simulink model "AprilTagPlant"  (R2024b)
settings: Solver=ode4  StartTime=0.0  StopTime=Tsim  FixedStep=0.005  RelTol=1e-3
values from neighbouring files (symbols this model uses):
  Caf = 20    [AprilTagVehicleSetup.m]
  Car = 20    [AprilTagVehicleSetup.m]
  circle_dir = 1    [AprilTagVehicleSetup.m]
  delta_corr_max_rad = deg2rad(20)    [AprilTagVehicleSetup.m]
  delta_max_rad = deg2rad(25)    [AprilTagVehicleSetup.m]
  delta_test_rad = deg2rad(8)    [AprilTagVehicleSetup.m]
  dist_psi_step_amp_rad = deg2rad(10)    [AprilTagVehicleSetup.m]
  dist_psi_step_time_s = 9.0    (= 9)    [AprilTagVehicleSetup.m]
  dist_x_step_amp_m = 0.10    (= 0.1)    [AprilTagVehicleSetup.m]
  dist_x_step_time_s = 5.0    (= 5)    [AprilTagVehicleSetup.m]
  dist_y_step_time_s = 7.0    (= 7)    [AprilTagVehicleSetup.m]
  Jz = 0.015    [AprilTagVehicleSetup.m]
  Kd_radius_pid = 0.0    (= 0)    [AprilTagVehicleSetup.m]
  Ki_radius_pid = 0.0    (= 0)    [AprilTagVehicleSetup.m]
  Kp_radius_pid = 0.6    [AprilTagVehicleSetup.m]
  L = 0.26    [AprilTagVehicleSetup.m]
  lf = 0.13    [AprilTagVehicleSetup.m]
  lr = 0.13    [AprilTagVehicleSetup.m]
  m = 1.5    [AprilTagVehicleSetup.m]
  noise_psi_std_rad = deg2rad(0.5)    [AprilTagVehicleSetup.m]
  noise_x_std_m = 0.005    [AprilTagVehicleSetup.m]
  noise_y_std_m = 0.005    [AprilTagVehicleSetup.m]
  psi0_rad = pi/2 - deg2rad(45)    [AprilTagVehicleSetup.m]
  psi_offset_max_rad = deg2rad(30)    [AprilTagVehicleSetup.m]
  r0_radps = 0.0    (= 0)    [AprilTagVehicleSetup.m]
  R_ref = 1.0    (= 1)    [AprilTagVehicleSetup.m]
  Ts_vision = 0.05    [AprilTagVehicleSetup.m]
  Vx_const = 1.0    (= 1)    [AprilTagVehicleSetup.m]
  Vy0 = 0.0    (= 0)    [AprilTagVehicleSetup.m]
  X0 = 0.4    [AprilTagVehicleSetup.m]
  xc = 0.0    (= 0)    [AprilTagVehicleSetup.m]
  Y0 = 0.0    (= 0)    [AprilTagVehicleSetup.m]
  yc = 0.0    (= 0)    [AprilTagVehicleSetup.m]
libraries: slpidlib x2
settings Model: Creator=mateu  LastModifiedBy=mateu

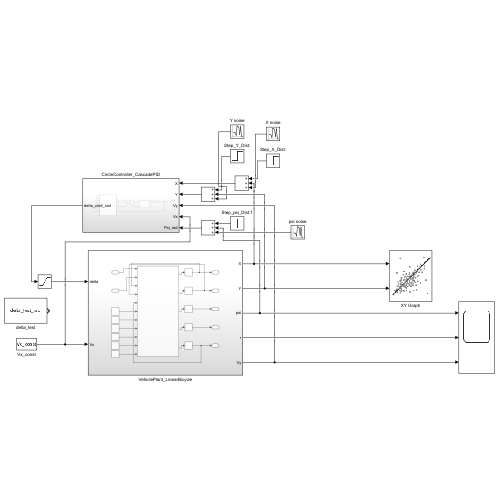
[thumbnail: Simulink's stored preview of the top-level diagram]
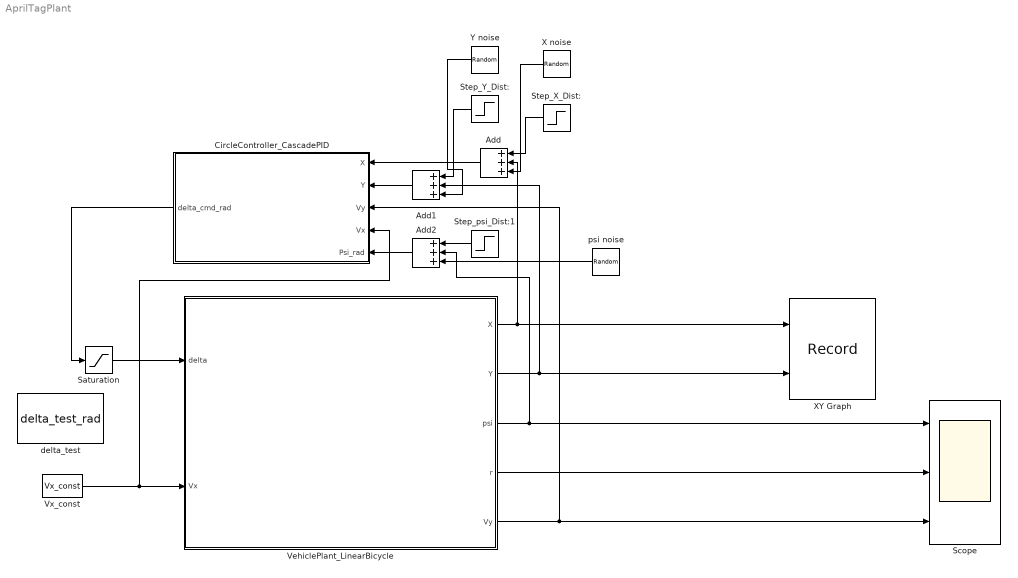
== system AprilTagPlant ==
  Add : Sum  Inputs=+++
  Add1 : Sum  Inputs=+++
  Add2 : Sum  Inputs=+++
  CircleController_CascadePID : Subsystem
  Saturation : Saturate  UpperLimit=delta_max_rad  LowerLimit=-delta_max_rad
  Scope : Scope  NumInputPorts=3
  Step_X_Dist: : Step  Time=dist_x_step_time_s  After=dist_x_step_amp_m  SampleTime=0
  Step_Y_Dist: : Step  Time=dist_y_step_time_s  After=dist_x_step_amp_m  SampleTime=0
  Step_psi_Dist:1 : Step  Time=dist_psi_step_time_s  After=dist_psi_step_amp_rad  SampleTime=0
  VehiclePlant_LinearBicycle : Subsystem
  Vx_const : Constant  Value=Vx_const
  X noise : RandomNumber  Variance=noise_x_std_m  SampleTime=Ts_vision
  XY Graph : Record  FileSettingsInternal="{\"entries\":[{\"content\":{\"excelSettings\":{\"content\":{},\"type\":\"Streamout.ExcelSettings\"}},\"type\":\"Streamout.FileSettingStorage\",\"uuid\":\"\"}],\"packageUris\":[\"http:\\/\\/schema.mathworks.com\\/mf0\\/streamout_blocks\\/R2020a\"],\"version\":\"1.0\"}"  Layout=[1 1]  SignalsInternal="{\"entries\":[{\"content\":{\"signals\":[{\"content\":{\"blockPath\":[],\"dimensions\":[1],\"domain\":\"\",\"lineColor\":\"#a2142f\",\"plots\":[ 1 ],\"port\":1,\"sid\":[\"\"],\"signalID\":1,\"signalName\":\"VehiclePlant_LinearBicycle:1\"},\"type\":\"RecordBlkView.Signal\",\"uuid\":\"\"},{\"content\":{\"blockPath\":[],\"dimensions\":[1],\"domain\":\"\",\"lineColor\":\"#139fff\",\"plots\":[ 1 ],\"port\":2,\"sid\":[\"\"],\"signalID\":2,\"signalName\":\"VehiclePlant_LinearBicycle:2\"},\"type\":\"RecordBlkView.Signal\",\"uuid\":\"\"}]},\"type\":\"RecordBlkView.InputSignals\",\"uuid\":\"\"}],\"packageUris\":[\"http:\\/\\/schema.mathworks.com\\/mf0\\/streamout_blocks\\/R2020a\"],\"version\":\"1.0\"}"  VisualizationBindings="{\"xyplotplugin\":{\"info\":[{\"series\":[{\"bindingParametersList\":[{\"parameter\":\"X-Axis\",\"signalID\":1,\"signalName\":\"VehiclePlant_LinearBicycle:1\"},{\"parameter\":\"Y-Axis\",\"signalID\":2,\"signalName\":\"VehiclePlant_LinearBicycle:2\"}],\"seriesID\":0}],\"subplotID\":1}]}}"  CompatibilityTag=XY
  Y noise : RandomNumber  Variance=noise_y_std_m  SampleTime=Ts_vision
  delta_test : Constant  Value=delta_test_rad
  psi noise : RandomNumber  Variance=noise_psi_std_rad  SampleTime=Ts_vision
  wires:
  Vx_const/1 -> CircleController_CascadePID/4(Vx), VehiclePlant_LinearBicycle/2(Vx)
  Saturation/1 -> VehiclePlant_LinearBicycle/1(delta)
  VehiclePlant_LinearBicycle/1(X) -> Add/2, XY Graph/1
  VehiclePlant_LinearBicycle/5(Vy) -> CircleController_CascadePID/3(Vy), Scope/3
  VehiclePlant_LinearBicycle/4(r) -> Scope/2
  VehiclePlant_LinearBicycle/3(psi) -> Add2/2, Scope/1
  VehiclePlant_LinearBicycle/2(Y) -> Add1/2, XY Graph/2
  CircleController_CascadePID/1(delta_cmd_rad) -> Saturation/1
  Step_X_Dist:/1 -> Add/1
  Add/1 -> CircleController_CascadePID/1(X)
  Add1/1 -> CircleController_CascadePID/2(Y)
  Step_Y_Dist:/1 -> Add1/1
  Step_psi_Dist:1/1 -> Add2/1
  Add2/1 -> CircleController_CascadePID/5(Psi_rad)
  X noise/1 -> Add/3
  Y noise/1 -> Add1/3
  psi noise/1 -> Add2/3

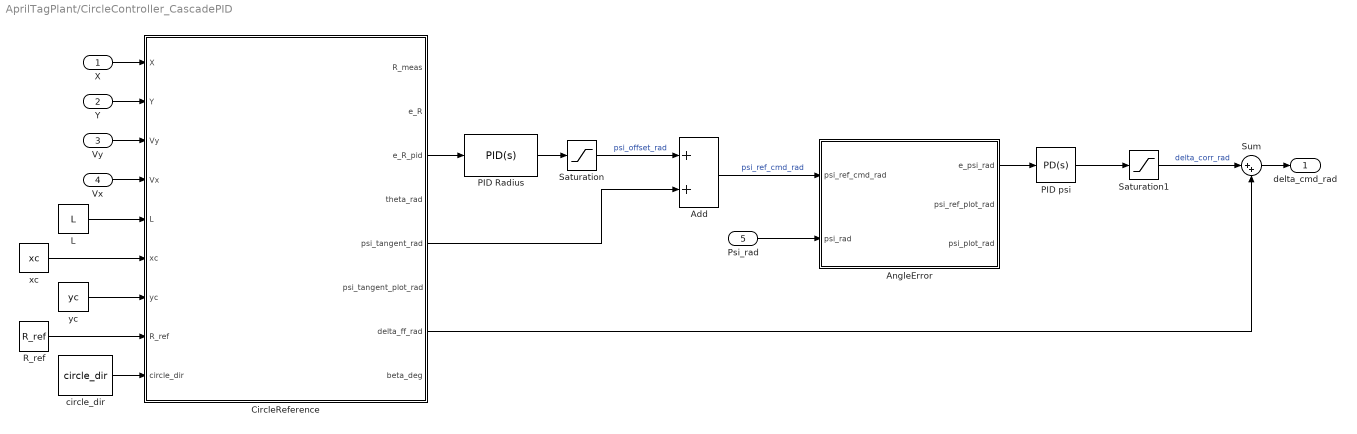
== system AprilTagPlant/CircleController_CascadePID ==
  X : Inport
  Y : Inport  Port=2
  Vy : Inport  Port=3
  Vx : Inport  Port=4
  Psi_rad : Inport  Port=5
  Add : Sum
  AngleError : MATLAB Function  TreatAsAtomicUnit=on
  CircleReference : MATLAB Function  TreatAsAtomicUnit=on
  L : Constant  Value=L
  PID Radius : slpidlib/PID Controller  Controller=PID  Form=Parallel  TimeDomain=Continuous-time  UseExternalTs=off  SampleTime=-1  IntegratorMethod=Forward Euler  FilterMethod=Forward Euler  ControllerParametersSource=internal  P=Kp_radius_pid  I=Ki_radius_pid  UseKiTs=off  D=Kd_radius_pid  UseExternalDerivativeSource=off  N=171.856773592637  UseFilter=on  TunerSelectOption=Transfer Function Based (PID Tuner App)  InitialConditionSource=internal  InitialConditionForIntegrator=0  InitialConditionForFilter=0  DifferentiatorICPrevScaledInput=0  ExternalReset=none  TrackingMode=off  Kt=1  LimitOutput=off  SatLimitsSource=internal  UpperSaturationLimit=inf  LowerSaturationLimit=-inf  LinearizeAsGain=on  AntiWindupMode=none  Kb=1  LimitIntegrator=off  UpperIntegratorSaturationLimit=inf  LowerIntegratorSaturationLimit=-inf  POutMin=[]  POutMax=[]  IOutMin=[]  IOutMax=[]  DOutMin=[]  DOutMax=[]  NOutMin=[]  NOutMax=[]  SumOutMin=[]  SumOutMax=[]  SaturationOutMin=[]  SaturationOutMax=[]  PParamMin=[]  PParamMax=[]  IParamMin=[]  IParamMax=[]  DParamMin=[]  DParamMax=[]  NParamMin=[]  NParamMax=[]  KbParamMin=[]  KbParamMax=[]  KtParamMin=[]  KtParamMax=[]  KbOutMin=[]  KbOutMax=[]  KtOutMin=[]  KtOutMax=[]  IntegratorOutMin=[]  IntegratorOutMax=[]  FilterOutMin=[]  FilterOutMax=[]  SumI1OutMin=[]  SumI1OutMax=[]  SumI2OutMin=[]  SumI2OutMax=[]  SumI3OutMin=[]  SumI3OutMax=[]  SumI4OutMin=[]  SumI4OutMax=[]  SumDOutMin=[]  SumDOutMax=[]  DifferentiatorOutMin=[]  DifferentiatorOutMax=[]  FilterDiffOutCoefMin=[]  FilterDiffOutCoefMax=[]  ReciprocalOutMin=[]  ReciprocalOutMax=[]  SumDenOutMin=[]  SumDenOutMax=[]  SumNumOutMin=[]  SumNumOutMax=[]  DivideOutMin=[]  DivideOutMax=[]  UdiffTsProdOutMin=[]  UdiffTsProdOutMax=[]  NTsProdOutMin=[]  NTsProdOutMax=[]  UintegralTsProdOutMin=[]  UintegralTsProdOutMax=[]  UngainTsProdOutMin=[]  UngainTsProdOutMax=[]  ClampingZeroOutDataTypeStr=Inherit: Inherit via back propagation  ClampingZeroOutMin=[]  ClampingZeroOutMax=[]  FilterDenConstantOutDataTypeStr=Inherit: Inherit via back propagation  FilterDenConstantOutMin=[]  FilterDenConstantOutMax=[]  PCopyOutDataTypeStr=Inherit: Inherit via back propagation  PCopyOutMin=[]  PCopyOutMax=[]  NCopyOutDataTypeStr=Inherit: Inherit via back propagation  NCopyOutMin=[]  NCopyOutMax=[]  IntegratorContinuousStateAttributes=''  IntegratorStateMustResolveToSignalObject=off  IntegratorRTWStateStorageClass=Auto  FilterContinuousStateAttributes=''  FilterStateMustResolveToSignalObject=off  FilterRTWStateStorageClass=Auto  ParallelPVariant=InternalParameters  IdealPVariant=Disabled  IVariant=InternalParameters  DVariant=InternalParameters  IntegratorVariant=Continuous  SatVariant=Disabled  AWVariant=Passthrough  PCopyVariant=Disabled  TRVariant=Disabled  FdbkBlocksVariant=Forward  IdealPFdbkVariant=Disabled  SatFdbkVariant=Disabled  DerivativeFilterVariant=ContFilter  NVariant=InternalParameters  NCopyVariant=Disabled  FilterICVariant=InternalICsFilter  IntegratorICVariant=InternalICs  ExternalResetVariant=Disabled  TRSumVariant=Passthrough  SumFdbkVariant=Disabled  SumVariant=Sum_PID  TsampFilterVariant=InternalTs  TsampNgainVariant=Passthrough  TsampIntegralVariant=Disabled_SignalSpec  ExternalSaturationOutDataTypeStr=Inherit: Same as second input  DerivativeSourceVariant=ErrorSignal  PreIntVariant=InternalPreInt
  PID psi : slpidlib/PID Controller  Controller=PD  Form=Parallel  TimeDomain=Continuous-time  UseExternalTs=off  SampleTime=-1  IntegratorMethod=Forward Euler  FilterMethod=Forward Euler  ControllerParametersSource=internal  P=-0.003865119901942  I=0  UseKiTs=off  D=-0.274008651407663  UseExternalDerivativeSource=off  N=184.215923888363  UseFilter=on  TunerSelectOption=Transfer Function Based (PID Tuner App)  InitialConditionSource=internal  InitialConditionForIntegrator=0  InitialConditionForFilter=0  DifferentiatorICPrevScaledInput=0  ExternalReset=none  TrackingMode=off  Kt=1  LimitOutput=off  SatLimitsSource=internal  UpperSaturationLimit=inf  LowerSaturationLimit=-inf  LinearizeAsGain=on  AntiWindupMode=none  Kb=1  LimitIntegrator=off  UpperIntegratorSaturationLimit=inf  LowerIntegratorSaturationLimit=-inf  POutMin=[]  POutMax=[]  IOutMin=[]  IOutMax=[]  DOutMin=[]  DOutMax=[]  NOutMin=[]  NOutMax=[]  SumOutMin=[]  SumOutMax=[]  SaturationOutMin=[]  SaturationOutMax=[]  PParamMin=[]  PParamMax=[]  IParamMin=[]  IParamMax=[]  DParamMin=[]  DParamMax=[]  NParamMin=[]  NParamMax=[]  KbParamMin=[]  KbParamMax=[]  KtParamMin=[]  KtParamMax=[]  KbOutMin=[]  KbOutMax=[]  KtOutMin=[]  KtOutMax=[]  IntegratorOutMin=[]  IntegratorOutMax=[]  FilterOutMin=[]  FilterOutMax=[]  SumI1OutMin=[]  SumI1OutMax=[]  SumI2OutMin=[]  SumI2OutMax=[]  SumI3OutMin=[]  SumI3OutMax=[]  SumI4OutMin=[]  SumI4OutMax=[]  SumDOutMin=[]  SumDOutMax=[]  DifferentiatorOutMin=[]  DifferentiatorOutMax=[]  FilterDiffOutCoefMin=[]  FilterDiffOutCoefMax=[]  ReciprocalOutMin=[]  ReciprocalOutMax=[]  SumDenOutMin=[]  SumDenOutMax=[]  SumNumOutMin=[]  SumNumOutMax=[]  DivideOutMin=[]  DivideOutMax=[]  UdiffTsProdOutMin=[]  UdiffTsProdOutMax=[]  NTsProdOutMin=[]  NTsProdOutMax=[]  UintegralTsProdOutMin=[]  UintegralTsProdOutMax=[]  UngainTsProdOutMin=[]  UngainTsProdOutMax=[]  ClampingZeroOutDataTypeStr=Inherit: Inherit via back propagation  ClampingZeroOutMin=[]  ClampingZeroOutMax=[]  FilterDenConstantOutDataTypeStr=Inherit: Inherit via back propagation  FilterDenConstantOutMin=[]  FilterDenConstantOutMax=[]  PCopyOutDataTypeStr=Inherit: Inherit via back propagation  PCopyOutMin=[]  PCopyOutMax=[]  NCopyOutDataTypeStr=Inherit: Inherit via back propagation  NCopyOutMin=[]  NCopyOutMax=[]  IntegratorContinuousStateAttributes=''  IntegratorStateMustResolveToSignalObject=off  IntegratorRTWStateStorageClass=Auto  FilterContinuousStateAttributes=''  FilterStateMustResolveToSignalObject=off  FilterRTWStateStorageClass=Auto  ParallelPVariant=InternalParameters  IdealPVariant=Disabled  IVariant=Disabled  DVariant=InternalParameters  IntegratorVariant=Disabled  SatVariant=Disabled  AWVariant=Disabled  PCopyVariant=Disabled  TRVariant=Disabled  FdbkBlocksVariant=Forward  IdealPFdbkVariant=Disabled  SatFdbkVariant=Disabled  DerivativeFilterVariant=ContFilter  NVariant=InternalParameters  NCopyVariant=Disabled  FilterICVariant=InternalICsFilter  IntegratorICVariant=Disabled  ExternalResetVariant=Disabled  TRSumVariant=Passthrough  SumFdbkVariant=Disabled  SumVariant=Sum_PD  TsampFilterVariant=InternalTs  TsampNgainVariant=Passthrough  TsampIntegralVariant=Disabled_SignalSpec  ExternalSaturationOutDataTypeStr=Inherit: Same as second input  DerivativeSourceVariant=ErrorSignal  PreIntVariant=InternalPreInt
  R_ref : Constant  Value=R_ref
  Saturation : Saturate  UpperLimit=psi_offset_max_rad  LowerLimit=-psi_offset_max_rad
  Saturation1 : Saturate  UpperLimit=delta_corr_max_rad  LowerLimit=-delta_corr_max_rad
  Sum : Sum  Inputs=|++
  circle_dir : Constant  Value=circle_dir
  xc : Constant  Value=xc
  yc : Constant  Value=yc
  delta_cmd_rad : Outport
  wires:
  X/1 -> CircleReference/1(X)
  Y/1 -> CircleReference/2(Y)
  Vy/1 -> CircleReference/3(Vy)
  Vx/1 -> CircleReference/4(Vx)
  yc/1 -> CircleReference/7(yc)
  R_ref/1 -> CircleReference/8(R_ref)
  circle_dir/1 -> CircleReference/9(circle_dir)
  L/1 -> CircleReference/5(L)
  xc/1 -> CircleReference/6(xc)
  CircleReference/3(e_R_pid) -> PID Radius/1
  PID Radius/1 -> Saturation/1
  Saturation/1 -> Add/1  "psi_offset_rad"
  CircleReference/5(psi_tangent_rad) -> Add/2
  Add/1 -> AngleError/1(psi_ref_cmd_rad)  "psi_ref_cmd_rad"
  Psi_rad/1 -> AngleError/2(psi_rad)
  AngleError/1(e_psi_rad) -> PID psi/1
  PID psi/1 -> Saturation1/1
  Saturation1/1 -> Sum/1  "delta_corr_rad"
  Sum/1 -> delta_cmd_rad/1
  CircleReference/7(delta_ff_rad) -> Sum/2

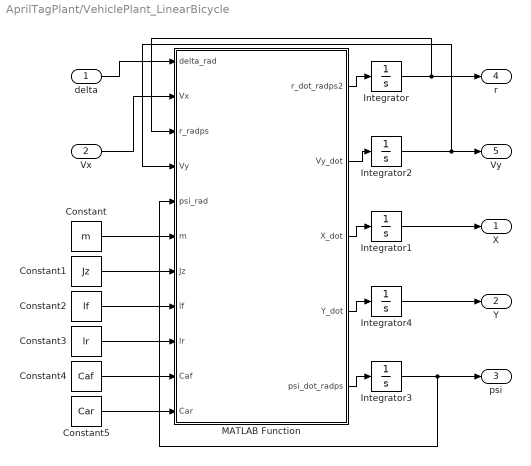
== system AprilTagPlant/VehiclePlant_LinearBicycle ==
  delta : Inport
  Vx : Inport  Port=2
  Constant : Constant  Value=m
  Constant1 : Constant  Value=Jz
  Constant2 : Constant  Value=lf
  Constant3 : Constant  Value=lr
  Constant4 : Constant  Value=Caf
  Constant5 : Constant  Value=Car
  Integrator : Integrator  InitialCondition=r0_radps
  Integrator1 : Integrator  InitialCondition=X0
  Integrator2 : Integrator  InitialCondition=Vy0
  Integrator3 : Integrator  InitialCondition=psi0_rad
  Integrator4 : Integrator  InitialCondition=Y0
  MATLAB Function : MATLAB Function  TreatAsAtomicUnit=on
  X : Outport
  Y : Outport  Port=2
  psi : Outport  Port=3
  r : Outport  Port=4
  Vy : Outport  Port=5
  wires:
  MATLAB Function/4(Y_dot) -> Integrator4/1
  MATLAB Function/1(r_dot_radps2) -> Integrator/1
  MATLAB Function/2(Vy_dot) -> Integrator2/1
  MATLAB Function/5(psi_dot_radps) -> Integrator3/1
  MATLAB Function/3(X_dot) -> Integrator1/1
  Integrator3/1 -> MATLAB Function/5(psi_rad), psi/1
  Integrator/1 -> MATLAB Function/3(r_radps), r/1
  Integrator1/1 -> X/1
  Integrator2/1 -> Vy/1, MATLAB Function/4(Vy)
  Vx/1 -> MATLAB Function/2(Vx)
  delta/1 -> MATLAB Function/1(delta_rad)
  Integrator4/1 -> Y/1
  Constant/1 -> MATLAB Function/6(m)
  Constant1/1 -> MATLAB Function/7(Jz)
  Constant2/1 -> MATLAB Function/8(lf)
  Constant3/1 -> MATLAB Function/9(lr)
  Constant4/1 -> MATLAB Function/10(Caf)
  Constant5/1 -> MATLAB Function/11(Car)

== matlab function AprilTagPlant/VehiclePlant_LinearBicycle/MATLAB Function ==
  data: delta_rad input; r_dot_radps2 output; Vx input; r_radps input; Vy input; psi_rad input; Vy_dot output; X_dot output; Y_dot output; psi_dot_radps output; m input; Jz input; lf input; lr input; Caf input; Car input
function [r_dot_radps2, Vy_dot, X_dot, Y_dot, psi_dot_radps] = BicycleDynamics(delta_rad, Vx, r_radps, Vy, psi_rad, m, Jz, lf, lr, Caf, Car)
% BicycleDynamics
%
% Konwencja:
% psi   - orientacja pojazdu / yaw [rad]
% r     - yaw rate = dpsi/dt [rad/s]
% delta - kąt skrętu kół [rad]
% Vy    - prędkość boczna w układzie pojazdu [m/s]
% Vx    - prędkość wzdłużna w układzie pojazdu [m/s]

% =========================
% Zabezpieczenia numeryczne
% =========================

Vx_min_local = 0.1;

if Vx < Vx_min_local
    Vx_eff = Vx_min_local;
else
    Vx_eff = Vx;
end

if Jz <= 0
    Jz_eff = 0.01;
else
    Jz_eff = Jz;
end

% =========================
% Kąty poślizgu opon
% =========================

alpha_f = atan((Vy + lf*r_radps) / Vx_eff) - delta_rad;
alpha_r = atan((Vy - lr*r_radps) / Vx_eff);

% =========================
% Liniowy model sił bocznych
% =========================

Fy_f = -Caf * alpha_f;
Fy_r = -Car * alpha_r;

% =========================
% Dynamika yaw i prędkości bocznej
% =========================

r_dot_radps2 = (lf * Fy_f * cos(delta_rad) - lr * Fy_r) / Jz_eff;

Vy_dot = (Fy_f * cos(delta_rad) + Fy_r) / m - r_radps * Vx;

% =========================
% Kinematyka globalna
% =========================

psi_dot_radps = r_radps;

X_dot = Vx * cos(psi_rad) - Vy * sin(psi_rad);
Y_dot = Vx * sin(psi_rad) + Vy * cos(psi_rad);

end

== matlab function AprilTagPlant/CircleController_CascadePID/CircleReference ==
  data: X input; R_meas output; Y input; Vy input; Vx input; L input; xc input; yc input; R_ref input; circle_dir input; e_R output; e_R_pid output; theta_rad output; psi_tangent_rad output; psi_tangent_plot_rad output; delta_ff_rad output; beta_deg output
function [R_meas, e_R, e_R_pid, theta_rad, psi_tangent_rad, psi_tangent_plot_rad, delta_ff_rad, beta_deg] = CircleReference(X, Y, Vy, Vx, L, xc, yc, R_ref, circle_dir)
% CircleReference
%
% Blok geometrii okręgu.
%
% Konwencja:
% theta - kąt położenia pojazdu względem środka okręgu, NIE yaw
% psi   - orientacja pojazdu / yaw
% delta - kąt skrętu kół
%
% Łańcuch fizyczny:
%
%   delta -> r -> psi -> X,Y -> R_meas
%
% delta nie zmienia promienia bezpośrednio. Najpierw zmienia yaw rate r,
% potem orientację psi, potem kierunek ruchu, a dopiero potem pozycję X,Y
% i promień R_meas.
%
% Dlatego w kaskadzie:
%
%   PID promienia: e_R -> psi_offset
%   PID psi:       e_psi -> delta_corr

dx = X - xc;
dy = Y - yc;

% Mierzony promień od środka okręgu
R_meas = sqrt(dx*dx + dy*dy);

% Klasyczny uchyb do wykresów:
% e_R > 0 -> auto jest za blisko środka
% e_R < 0 -> auto jest za daleko od środka
e_R = R_ref - R_meas;

% Sygnał na PID promienia.
% Znak uwzględnia kierunek jazdy po okręgu.
e_R_pid = -circle_dir * e_R;

% Kąt położenia na okręgu
% To NIE jest orientacja auta.
theta_rad = atan2(dy, dx);

% Kierunek styczny do okręgu
psi_tangent_rad = theta_rad + circle_dir*pi/2;

% Do wykresu zawijamy do -pi..pi
psi_tangent_plot_rad = atan2(sin(psi_tangent_rad), cos(psi_tangent_rad));

% Feedforward skrętu wynikający z geometrii modelu rowerowego
% delta_ff = atan(L/R)
delta_ff_rad = circle_dir * atan(L / R_ref);

% Diagnostyka poślizgu bocznego
beta_rad = atan2(Vy, Vx);
beta_deg = beta_rad * 180/pi;

end

== matlab function AprilTagPlant/CircleController_CascadePID/AngleError ==
  data: psi_ref_cmd_rad input; e_psi_rad output; psi_rad input; psi_ref_plot_rad output; psi_plot_rad output
function [e_psi_rad, psi_ref_plot_rad, psi_plot_rad] = AngleError(psi_ref_cmd_rad, psi_rad)
% AngleError
%
% Liczy uchyb orientacji:
%
%   e_psi = psi_ref_cmd - psi
%
% z zawinięciem do -pi..pi, żeby uniknąć skoku np. 179 deg -> -179 deg.
%
% PID nie musi mieć wyjścia w tej samej jednostce co wejście.
% Tutaj:
%
%   e_psi_rad -> PID_Psi -> delta_corr_rad
%
% czyli uchyb orientacji [rad] jest przeliczany przez wzmocnienia PID
% na korektę skrętu kół [rad].
%
% To jest analogiczne do:
%
%   uchyb temperatury [degC] -> PID -> moc grzałki [%]

e_psi_rad = atan2(sin(psi_ref_cmd_rad - psi_rad), cos(psi_ref_cmd_rad - psi_rad));

psi_ref_plot_rad = atan2(sin(psi_ref_cmd_rad), cos(psi_ref_cmd_rad));
psi_plot_rad     = atan2(sin(psi_rad),         cos(psi_rad));

end
